simulink model "Project2_2016b"  (R2016b)
settings: Solver=VariableStepAuto  StartTime=0.0  StopTime=10.0  RelTol=1e-3
values from neighbouring files (symbols this model uses):
  C = 1e-3    (= 0.001)    [init.m]
  Kd = 2    [init.m]
  Kq = 2    [init.m]
  L = 5e-6    (= 5e-06)    [init.m]
  lambda_m = 0.266    [init.m]
  Ld = 0.8e-3    (= 0.0008)    [init.m]
  Lq = 1.0e-3    (= 0.001)    [init.m]
  P = 8    [init.m]
  R = 0.01    [init.m]
  rs = 0.07    [init.m]
  V_batt = 600    [init.m]
libraries: simulink x1
settings Model: Creator=wasynczu  LastModifiedBy=wasynczu
settings DataIOCC: ReturnWorkspaceOutputs=on
settings SFSimCC: SimUseLocalCustomCode=on
settings RTWCC: RTWUseLocalCustomCode=on

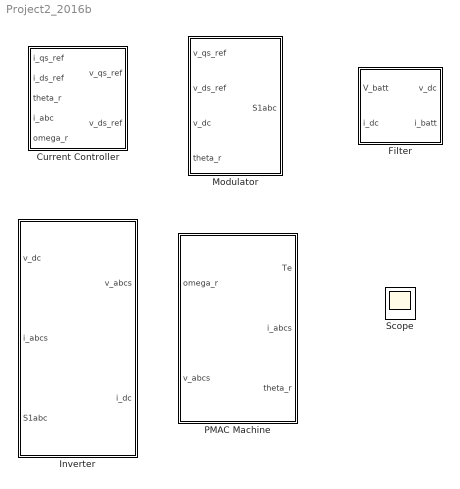
== system Project2_2016b ==
  Current Controller : Subsystem
  Filter : Subsystem
  Inverter : Subsystem
  Modulator : Subsystem
  PMAC Machine : Subsystem
  Scope : Scope

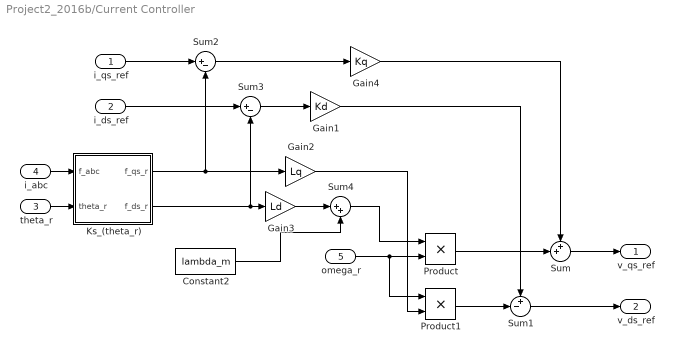
== system Project2_2016b/Current Controller ==
  i_qs_ref : Inport
  i_ds_ref : Inport  Port=2
  theta_r : Inport  Port=3
  i_abc : Inport  Port=4
  omega_r : Inport  Port=5
  Constant2 : Constant  Value=lambda_m
  Gain1 : Gain  Gain=Kd
  Gain2 : Gain  Gain=Lq
  Gain3 : Gain  Gain=Ld
  Gain4 : Gain  Gain=Kq
  Ks_(theta_r) : Subsystem
  Product : Product
  Product1 : Product
  Sum : Sum  Inputs=++|
  Sum1 : Sum  Inputs=+-|
  Sum2 : Sum  Inputs=|+-
  Sum3 : Sum  Inputs=|+-
  Sum4 : Sum  Inputs=|++
  v_qs_ref : Outport
  v_ds_ref : Outport  Port=2
  wires:
  Gain4/1 -> Sum/1
  Constant2/1 -> Sum4/2
  Sum4/1 -> Product/1
  Gain3/1 -> Sum4/1
  Gain2/1 -> Product1/2
  Ks_(theta_r)/2(f_ds_r) -> Gain3/1, Sum3/2
  Ks_(theta_r)/1(f_qs_r) -> Sum2/2, Gain2/1
  i_abc/1 -> Ks_(theta_r)/1(f_abc)
  i_qs_ref/1 -> Sum2/1
  i_ds_ref/1 -> Sum3/1
  Gain1/1 -> Sum1/1
  Sum2/1 -> Gain4/1
  Sum3/1 -> Gain1/1
  Sum1/1 -> v_ds_ref/1
  Product1/1 -> Sum1/2
  Sum/1 -> v_qs_ref/1
  omega_r/1 -> Product/2, Product1/1
  Product/1 -> Sum/2
  theta_r/1 -> Ks_(theta_r)/2(theta_r)

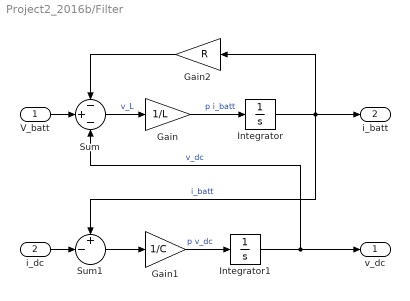
== system Project2_2016b/Filter ==
  V_batt : Inport
  i_dc : Inport  Port=2
  Gain : Gain  Gain=1/L
  Gain1 : Gain  Gain=1/C
  Gain2 : Gain  Gain=R
  Integrator : Integrator
  Integrator1 : Integrator  InitialCondition=V_batt
  Sum : Sum  Inputs=-+-
  Sum1 : Sum  Inputs=+-|
  v_dc : Outport
  i_batt : Outport  Port=2
  wires:
  Gain1/1 -> Integrator1/1  "p v_dc"
  Gain2/1 -> Sum/1
  V_batt/1 -> Sum/2
  Integrator1/1 -> Sum/3, v_dc/1  "v_dc"
  Sum1/1 -> Gain1/1
  i_dc/1 -> Sum1/2
  Integrator/1 -> Sum1/1, i_batt/1, Gain2/1  "i_batt"
  Gain/1 -> Integrator/1  "p i_batt"
  Sum/1 -> Gain/1  "v_L"

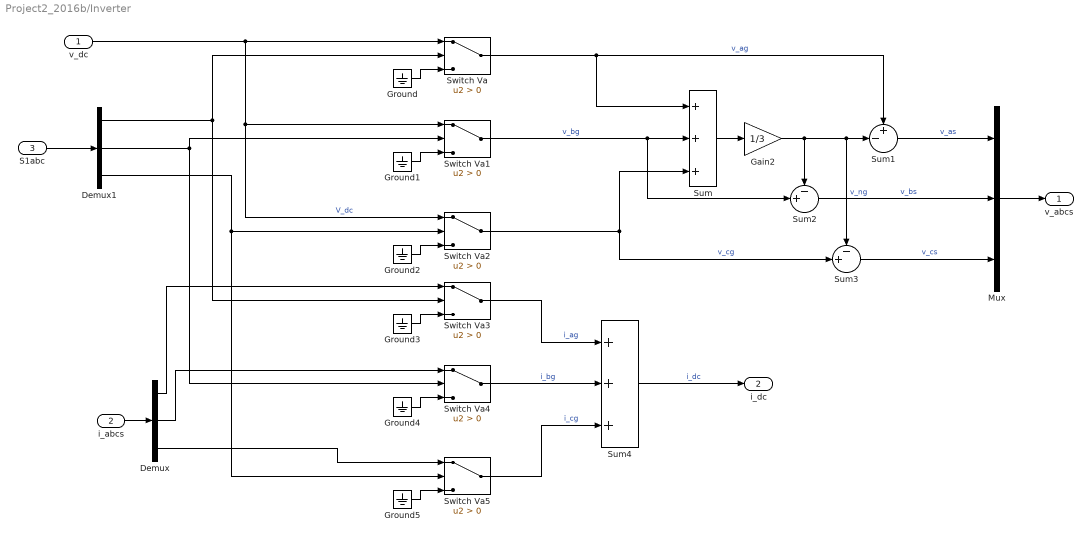
== system Project2_2016b/Inverter ==
  v_dc : Inport
  i_abcs : Inport  Port=2
  S1abc : Inport  Port=3
  Demux : Demux  Outputs=3
  Demux1 : Demux  Outputs=3
  Gain2 : Gain  Gain=1/3
  Ground{,1..5} (6 alike) : Ground
  Mux : Mux  Inputs=3
  Sum : Sum  Inputs=+++
  Sum1 : Sum  Inputs=+-|
  Sum2 : Sum  Inputs=-+|
  Sum3 : Sum  Inputs=-+|
  Sum4 : Sum  Inputs=+++
  Switch Va{,1..5} (6 alike) : Switch  Criteria=u2 > Threshold
  v_abcs : Outport
  i_dc : Outport  Port=2
  wires:
  S1abc/1 -> Demux1/1
  Sum1/1 -> Mux/1  "v_as"
  Mux/1 -> v_abcs/1
  Demux/1 -> Switch Va3/1
  i_abcs/1 -> Demux/1
  Demux/3 -> Switch Va5/1
  Sum4/1 -> i_dc/1  "i_dc"
  Demux/2 -> Switch Va4/1
  Sum3/1 -> Mux/3  "v_cs"
  Sum2/1 -> Mux/2  "v_bs"
  Switch Va5/1 -> Sum4/3  "i_cg"
  Switch Va4/1 -> Sum4/2  "i_bg"
  Switch Va3/1 -> Sum4/1  "i_ag"
  Ground5/1 -> Switch Va5/3
  Ground4/1 -> Switch Va4/3
  Ground3/1 -> Switch Va3/3
  Gain2/1 -> Sum3/1, Sum1/2, Sum2/1  "v_ng"
  Sum/1 -> Gain2/1
  Switch Va2/1 -> Sum3/2, Sum/3  "v_cg"
  Switch Va1/1 -> Sum2/2, Sum/2  "v_bg"
  Switch Va/1 -> Sum1/1, Sum/1  "v_ag"
  Demux1/3 -> Switch Va5/2, Switch Va2/2
  Demux1/2 -> Switch Va4/2, Switch Va1/2
  Demux1/1 -> Switch Va3/2, Switch Va/2
  v_dc/1 -> Switch Va/1, Switch Va2/1, Switch Va1/1  "V_dc"
  Ground2/1 -> Switch Va2/3
  Ground1/1 -> Switch Va1/3
  Ground/1 -> Switch Va/3

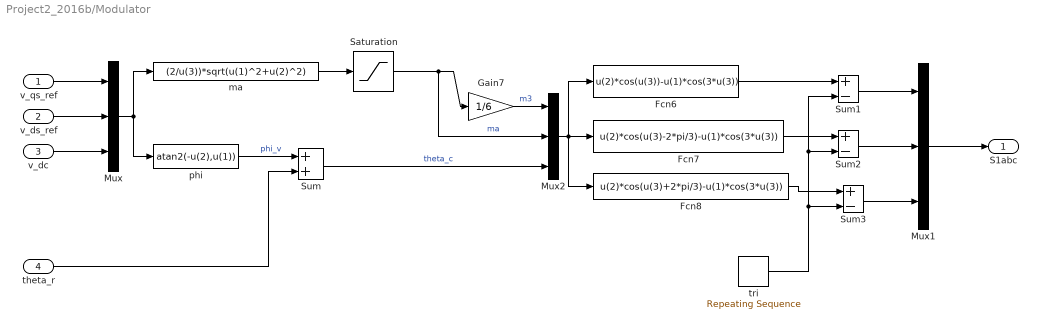
== system Project2_2016b/Modulator ==
  v_qs_ref : Inport
  v_ds_ref : Inport  Port=2
  v_dc : Inport  Port=3
  theta_r : Inport  Port=4
  Fcn6 : Fcn  Expr=u(2)*cos(u(3))-u(1)*cos(3*u(3))
  Fcn7 : Fcn  Expr=u(2)*cos(u(3)-2*pi/3)-u(1)*cos(3*u(3))
  Fcn8 : Fcn  Expr=u(2)*cos(u(3)+2*pi/3)-u(1)*cos(3*u(3))
  Gain7 : Gain  Gain=1/6
  Mux : Mux  Inputs=3
  Mux1 : Mux  Inputs=3
  Mux2 : Mux  Inputs=3
  Saturation : Saturate  UpperLimit=2/sqrt(3)  LowerLimit=0
  Sum : Sum
  Sum1 : Sum  Inputs=+-
  Sum2 : Sum  Inputs=+-
  Sum3 : Sum  Inputs=+-
  ma : Fcn  Expr=(2/u(3))*sqrt(u(1)^2+u(2)^2)
  phi : Fcn  Expr=atan2(-u(2),u(1))
  tri : simulink/Sources/Repeating Sequence  rep_seq_t=[0 1/40000 1/20000 3/40000 1/10000]*0.5  rep_seq_y=[0 1 0 -1 0]
  S1abc : Outport
  wires:
  Mux1/1 -> S1abc/1
  Sum1/1 -> Mux1/1
  theta_r/1 -> Sum/2
  Saturation/1 -> Mux2/2, Gain7/1  "ma"
  ma/1 -> Saturation/1
  Fcn8/1 -> Sum3/1
  Fcn7/1 -> Sum2/1
  Fcn6/1 -> Sum1/1
  Gain7/1 -> Mux2/1  "m3"
  Mux2/1 -> Fcn8/1, Fcn7/1, Fcn6/1
  Sum/1 -> Mux2/3  "theta_c"
  phi/1 -> Sum/1  "phi_v"
  Mux/1 -> phi/1, ma/1
  v_dc/1 -> Mux/3
  v_ds_ref/1 -> Mux/2
  v_qs_ref/1 -> Mux/1
  Sum3/1 -> Mux1/3
  Sum2/1 -> Mux1/2
  tri/1 -> Sum3/2, Sum1/2, Sum2/2

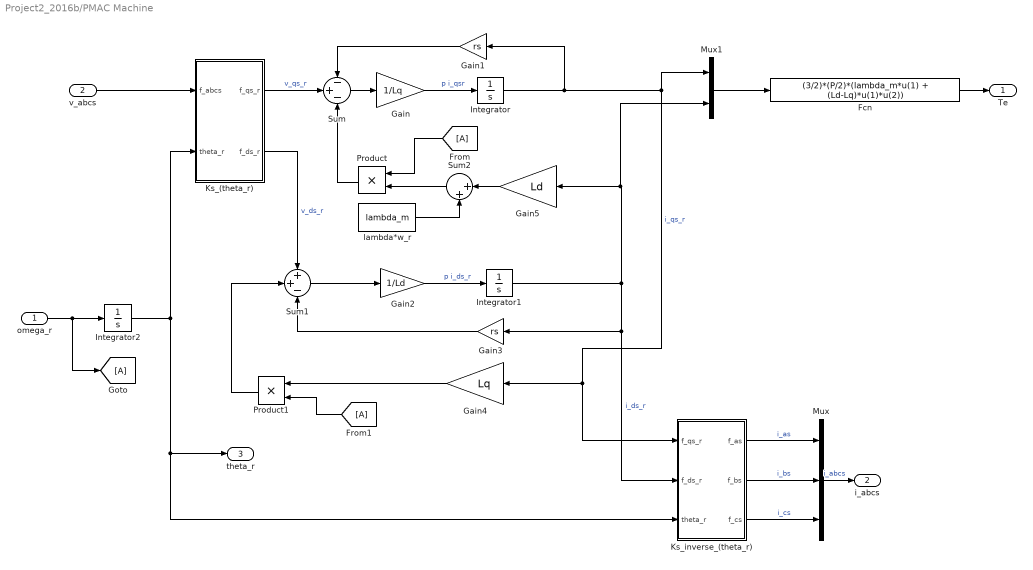
== system Project2_2016b/PMAC Machine ==
  omega_r : Inport
  v_abcs : Inport  Port=2
  Fcn : Fcn  Expr=(3/2)*(P/2)*(lambda_m*u(1) + (Ld-Lq)*u(1)*u(2))
  Gain : Gain  Gain=1/Lq
  Gain1 : Gain  Gain=rs
  Gain2 : Gain  Gain=1/Ld
  Gain3 : Gain  Gain=rs
  Gain4 : Gain  Gain=Lq
  Gain5 : Gain  Gain=Ld
  Integrator : Integrator
  Integrator1 : Integrator
  Integrator2 : Integrator
  Ks_(theta_r) : Subsystem
  Ks_inverse_(theta_r) : Subsystem
  Mux : Mux  Inputs=3
  Mux1 : Mux  Inputs=2
  Product : Product
  Product1 : Product
  Sum : Sum  Inputs=-+-
  Sum1 : Sum  Inputs=++-
  Sum2 : Sum  Inputs=|++
  lambda*w_r : Constant  Value=lambda_m
  Te : Outport
  i_abcs : Outport  Port=2
  theta_r : Outport  Port=3
  wires:
  Mux1/1 -> Fcn/1
  [A] -> Product1/2
  Product1/1 -> Sum1/2
  Gain4/1 -> Product1/1
  [A] -> Product/1
  Product/1 -> Sum/3
  Gain1/1 -> Sum/1
  Sum2/1 -> Product/2
  lambda*w_r/1 -> Sum2/2
  Gain5/1 -> Sum2/1
  omega_r/1 -> Integrator2/1, [A]
  v_abcs/1 -> Ks_(theta_r)/1(f_abcs)
  Mux/1 -> i_abcs/1  "i_abcs"
  Fcn/1 -> Te/1
  Ks_inverse_(theta_r)/3(f_cs) -> Mux/3  "i_cs"
  Ks_inverse_(theta_r)/2(f_bs) -> Mux/2  "i_bs"
  Ks_inverse_(theta_r)/1(f_as) -> Mux/1  "i_as"
  Integrator2/1 -> theta_r/1, Ks_inverse_(theta_r)/3(theta_r), Ks_(theta_r)/2(theta_r)
  Gain3/1 -> Sum1/3
  Integrator1/1 -> Ks_inverse_(theta_r)/2(f_ds_r), Gain3/1, Gain5/1, Mux1/2  "i_ds_r"
  Gain2/1 -> Integrator1/1  "p i_ds_r"
  Sum1/1 -> Gain2/1
  Integrator/1 -> Gain1/1, Ks_inverse_(theta_r)/1(f_qs_r), Gain4/1, Mux1/1  "i_qs_r"
  Gain/1 -> Integrator/1  "p i_qsr"
  Sum/1 -> Gain/1
  Ks_(theta_r)/1(f_qs_r) -> Sum/2  "v_qs_r"
  Ks_(theta_r)/2(f_ds_r) -> Sum1/1  "v_ds_r"

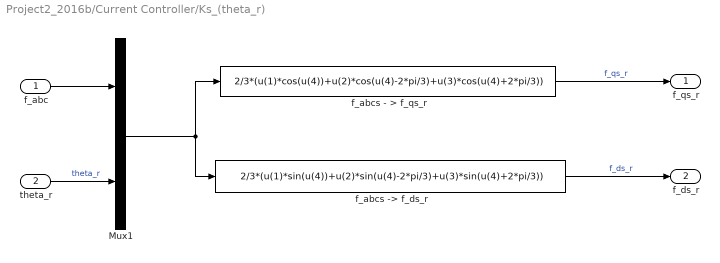
== system Project2_2016b/Current Controller/Ks_(theta_r) ==
  f_abc : Inport
  theta_r : Inport  Port=2
  Mux1 : Mux  Inputs=2
  f_abcs - > f_qs_r : Fcn  Expr=2/3*(u(1)*cos(u(4))+u(2)*cos(u(4)-2*pi/3)+u(3)*cos(u(4)+2*pi/3))
  "f_abcs -> f_ds_r" : Fcn  Expr=2/3*(u(1)*sin(u(4))+u(2)*sin(u(4)-2*pi/3)+u(3)*sin(u(4)+2*pi/3))
  f_qs_r : Outport
  f_ds_r : Outport  Port=2
  wires:
  theta_r/1 -> Mux1/2  "theta_r"
  Mux1/1 -> f_abcs - > f_qs_r/1, "f_abcs -> f_ds_r"/1
  f_abcs - > f_qs_r/1 -> f_qs_r/1  "f_qs_r"
  f_abc/1 -> Mux1/1
  "f_abcs -> f_ds_r"/1 -> f_ds_r/1  "f_ds_r"

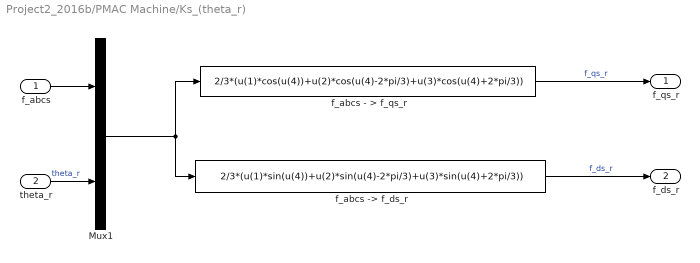
== system Project2_2016b/PMAC Machine/Ks_(theta_r) ==
  f_abcs : Inport
  theta_r : Inport  Port=2
  Mux1 : Mux  Inputs=2
  f_abcs - > f_qs_r : Fcn  Expr=2/3*(u(1)*cos(u(4))+u(2)*cos(u(4)-2*pi/3)+u(3)*cos(u(4)+2*pi/3))
  "f_abcs -> f_ds_r" : Fcn  Expr=2/3*(u(1)*sin(u(4))+u(2)*sin(u(4)-2*pi/3)+u(3)*sin(u(4)+2*pi/3))
  f_qs_r : Outport
  f_ds_r : Outport  Port=2
  wires:
  theta_r/1 -> Mux1/2  "theta_r"
  Mux1/1 -> f_abcs - > f_qs_r/1, "f_abcs -> f_ds_r"/1
  f_abcs - > f_qs_r/1 -> f_qs_r/1  "f_qs_r"
  f_abcs/1 -> Mux1/1
  "f_abcs -> f_ds_r"/1 -> f_ds_r/1  "f_ds_r"

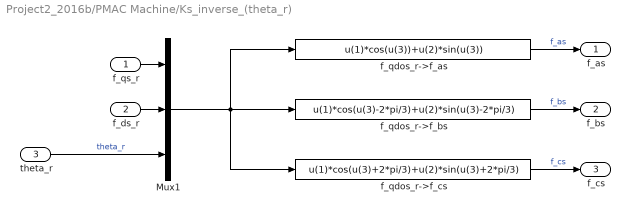
== system Project2_2016b/PMAC Machine/Ks_inverse_(theta_r) ==
  f_qs_r : Inport
  f_ds_r : Inport  Port=2
  theta_r : Inport  Port=3
  Mux1 : Mux  Inputs=3
  f_qdos_r->f_as : Fcn  Expr=u(1)*cos(u(3))+u(2)*sin(u(3))
  f_qdos_r->f_bs : Fcn  Expr=u(1)*cos(u(3)-2*pi/3)+u(2)*sin(u(3)-2*pi/3)
  f_qdos_r->f_cs : Fcn  Expr=u(1)*cos(u(3)+2*pi/3)+u(2)*sin(u(3)+2*pi/3)
  f_as : Outport
  f_bs : Outport  Port=2
  f_cs : Outport  Port=3
  wires:
  f_qdos_r->f_cs/1 -> f_cs/1  "f_cs"
  f_qdos_r->f_bs/1 -> f_bs/1  "f_bs"
  f_ds_r/1 -> Mux1/2
  f_qs_r/1 -> Mux1/1
  f_qdos_r->f_as/1 -> f_as/1  "f_as"
  Mux1/1 -> f_qdos_r->f_cs/1, f_qdos_r->f_bs/1, f_qdos_r->f_as/1
  theta_r/1 -> Mux1/3  "theta_r"
